simulink model "Project1_Option1_stiffness"  (R2024b)
settings: Solver=ode1  StartTime=0.0  StopTime=25  FixedStep=0.1  RelTol=1e-3
values from neighbouring files (symbols this model uses):
  b1 = 1    [Part2_Option1_Code.m]    (also in Part2_Option3_Code.m; Part2_option2_code.m)
  b2 = 1    [Part2_Option1_Code.m]    (also in Part2_Option3_Code.m; Part2_option2_code.m)
  J1 = 100    [Part2_Option1_Code.m]    (also in Part2_Option3_Code.m; Part2_option2_code.m; Project1_Part1_Code_revision_1.m = [100, 0.01]; Project1_Part1_Code_revision_current.m = [100, 0.01])
  J2 = 1    [Part2_Option1_Code.m]    (also in Part2_Option3_Code.m; Part2_option2_code.m)
  omega_init = [10,0]    [Part2_Option1_Code.m]    (also in Part2_Option3_Code.m; Part2_option2_code.m; Project1_Part1_Code_revision_1.m; Project1_Part1_Code_revision_current.m)
  tau = [0, 100]    [Part2_option2_code.m]    (also in Project1_Part1_Code_revision_1.m; Project1_Part1_Code_revision_current.m)
  theta0 = 0    [P1.m]    (also in Part2_Option1_Code.m; Part2_Option3_Code.m; Part2_option2_code.m; Project1_Part1_Code_revision_1.m)
  torque_mode = [1,0]    [P1.m]    (also in Part2_Option1_Code.m = [0,1]; Part2_Option3_Code.m = [0,1]; Part2_option2_code.m = [0,1]; Project1_Part1_Code_revision_1.m = [0,1])
  w_freq = [0.1, 100]    [Part2_Option1_Code.m]    (also in Part2_Option3_Code.m; Part2_option2_code.m; Project1_Part1_Code_revision_current.m)
undefined symbols (not defined in the file or in its folder): k
settings Model: Creator=jacobcody  LastModifiedBy=jacobcody

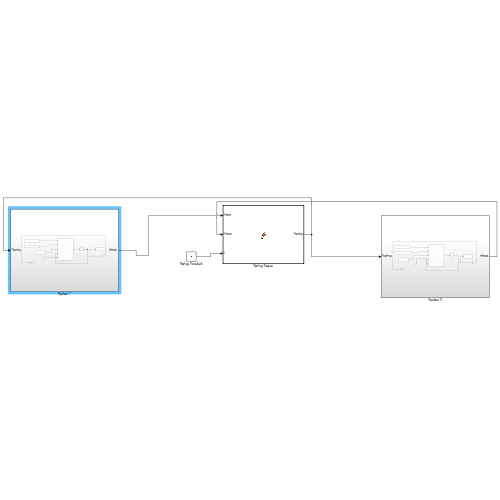
[thumbnail: Simulink's stored preview of the top-level diagram]
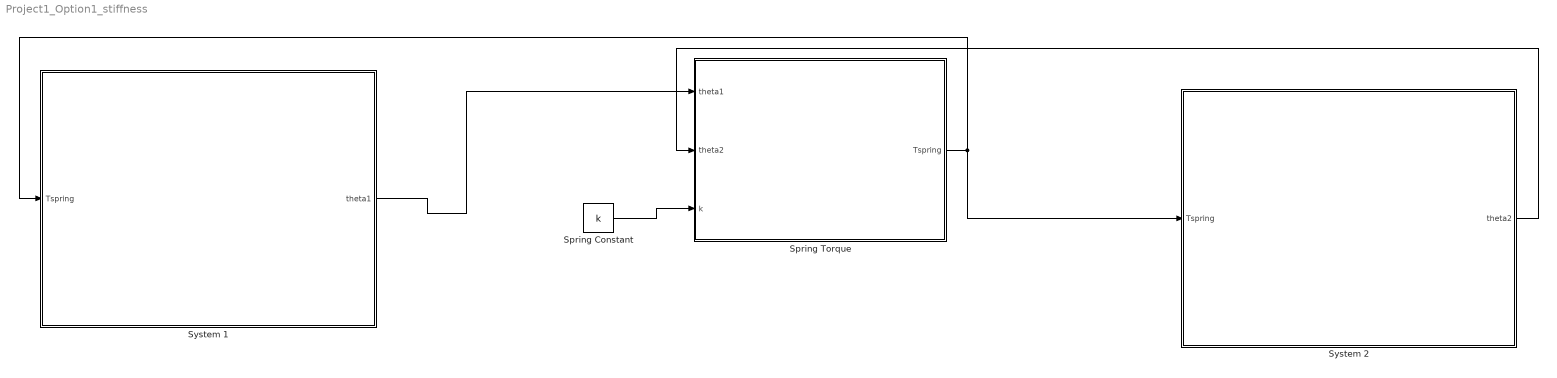
== system Project1_Option1_stiffness ==
  Spring Constant : Constant  Value=k
  Spring Torque : MATLAB Function  TreatAsAtomicUnit=on
  System 1 : Subsystem
  System 2 : Subsystem
  wires:
  System 2/1(theta2) -> Spring Torque/2(theta2)
  Spring Constant/1 -> Spring Torque/3(k)
  System 1/1(theta1) -> Spring Torque/1(theta1)
  Spring Torque/1(Tspring) -> System 2/1(Tspring), System 1/1(Tspring)

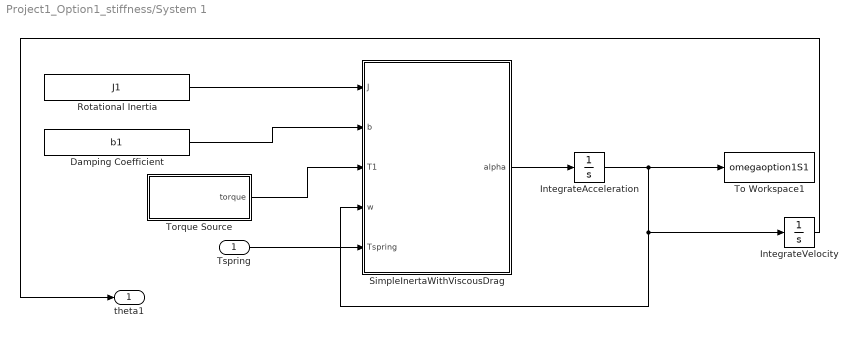
== system Project1_Option1_stiffness/System 1 ==
  Tspring : Inport
  Damping Coefficient : Constant  Value=b1
  IntegrateAcceleration : Integrator  InitialCondition=omega_init
  IntegrateVelocity : Integrator  InitialCondition=theta0
  Rotational Inertia : Constant  Value=J1
  SimpleInertaWithViscousDrag : MATLAB Function  TreatAsAtomicUnit=on
  To Workspace1 : ToWorkspace  VariableName=omegaoption1S1  SaveFormat=Timeseries  SampleTime=-1
  Torque Source : Subsystem
  theta1 : Outport
  wires:
  Tspring/1 -> SimpleInertaWithViscousDrag/5(Tspring)
  IntegrateAcceleration/1 -> IntegrateVelocity/1, SimpleInertaWithViscousDrag/4(w), To Workspace1/1
  IntegrateVelocity/1 -> theta1/1
  Damping Coefficient/1 -> SimpleInertaWithViscousDrag/2(b)
  Rotational Inertia/1 -> SimpleInertaWithViscousDrag/1(J)
  SimpleInertaWithViscousDrag/1(alpha) -> IntegrateAcceleration/1
  Torque Source/1(torque) -> SimpleInertaWithViscousDrag/3(T1)

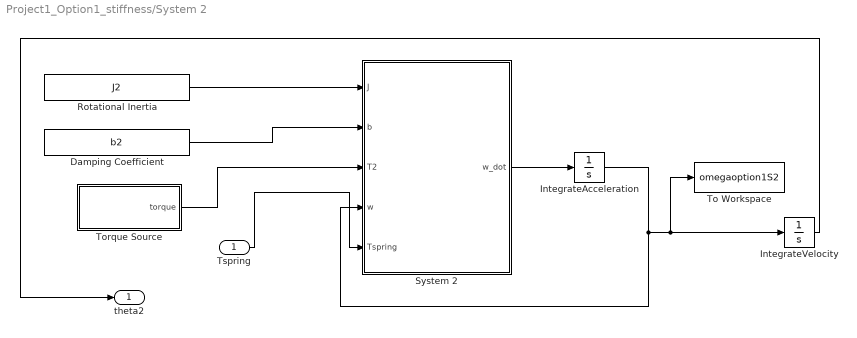
== system Project1_Option1_stiffness/System 2 ==
  Tspring : Inport
  Damping Coefficient : Constant  Value=b2
  IntegrateAcceleration : Integrator  InitialCondition=omega_init
  IntegrateVelocity : Integrator  InitialCondition=theta0
  Rotational Inertia : Constant  Value=J2
  System 2 : MATLAB Function  TreatAsAtomicUnit=on
  To Workspace : ToWorkspace  VariableName=omegaoption1S2  SaveFormat=Timeseries  SampleTime=-1
  Torque Source : Subsystem
  theta2 : Outport
  wires:
  Tspring/1 -> System 2/5(Tspring)
  IntegrateAcceleration/1 -> IntegrateVelocity/1, To Workspace/1, System 2/4(w)
  IntegrateVelocity/1 -> theta2/1
  Damping Coefficient/1 -> System 2/2(b)
  Rotational Inertia/1 -> System 2/1(J)
  System 2/1(w_dot) -> IntegrateAcceleration/1
  Torque Source/1(torque) -> System 2/3(T2)

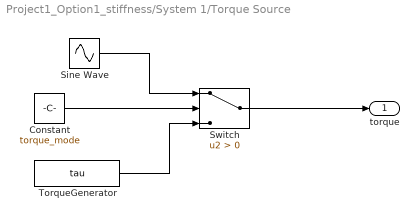
== system Project1_Option1_stiffness/System 1/Torque Source ==
  Constant : Constant  Value=torque_mode
  Sine Wave : Sin  Frequency=w_freq  SampleTime=0
  Switch : Switch  Criteria=u2 > Threshold  SaturateOnIntegerOverflow=off  InputSameDT=off
  TorqueGenerator : Constant  Value=tau
  torque : Outport
  wires:
  Switch/1 -> torque/1
  Sine Wave/1 -> Switch/1
  TorqueGenerator/1 -> Switch/3
  Constant/1 -> Switch/2

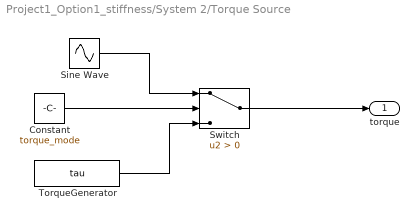
== system Project1_Option1_stiffness/System 2/Torque Source ==
  Constant : Constant  Value=torque_mode
  Sine Wave : Sin  Frequency=w_freq  SampleTime=0
  Switch : Switch  Criteria=u2 > Threshold  SaturateOnIntegerOverflow=off  InputSameDT=off
  TorqueGenerator : Constant  Value=tau
  torque : Outport
  wires:
  Switch/1 -> torque/1
  Sine Wave/1 -> Switch/1
  TorqueGenerator/1 -> Switch/3
  Constant/1 -> Switch/2

== matlab function Project1_Option1_stiffness/Spring Torque ==
  data: theta1 input; Tspring output; theta2 input; k input
function Tspring = fcn(theta1, theta2, k)
Tspring= k*(theta1-theta2);

== matlab function Project1_Option1_stiffness/System 1/SimpleInertaWithViscousDrag ==
  data: J input; b input; T1 input; w input; alpha output; Tspring input
function alpha = fcn(J, b, T1, w, Tspring)
alpha = ((T1-Tspring) - w * b)/J;

== matlab function Project1_Option1_stiffness/System 2/System 2 ==
  data: J input; b input; T2 input; w input; w_dot output; Tspring input
function w_dot = fcn(J, b, T2, w, Tspring)
w_dot = ((T2-Tspring) - w * b)/J;
